simulink model "hoverSim_pid_RL"  (R2025b)
settings: Solver=ode45  StartTime=0.0  StopTime=30  RelTol=1e-3  AbsTol=1e-3  EnableMultiTasking=on
values from neighbouring files (symbols this model uses):
  A = [0 0 0 1 0 0 ... (first row only)    [setupHover.m]
  B = [0     0     0     0 ... (first row only)    [setupHover.m]
  C = [1 0 0 0 0 0 ... (first row only)    [setupHover.m]
  CMD_RATE_LIMIT = 60 * pi/180    (= 1.0471975512)    [setupHover.m]
  D = zeros(3,4)    [setupHover.m]
  K = [ 1  1  0 ... (first row only)    [setupHover.m]
  V_bias = 2.0    (= 2)    [setupHover.m]
  VMAX_AMP = 24    [setupHover.m]
  wcf = 2 * pi * 20    (= 125.663706144)    [setupHover.m]
  zetaf = 0.6    [setupHover.m]
undefined symbols (not defined in the file or in its folder): X, Y, Z
libraries: sm_lib x30, rllib x18, simulink_extras x17, slpidlib x6, nesl_utility x4, simulink x2
(part 1 of 3)
settings Model: Creator=2922887  LastModifiedBy=oleruus
settings SolverCC: AutoScaleAbsTol=off  AlgebraicLoopSolver=TrustRegion
settings DataIOCC: LimitDataPoints=on  MaxDataPoints=10000
settings OptimizationCC: LifeSpan=inf
settings DebuggingCC: UnconnectedInputMsg=warning  UnconnectedOutputMsg=warning  UnconnectedLineMsg=warning  AllowSymbolicDim=off  SFUnexpectedBacktrackingDiag=warning  SFNoUnconditionalDefaultTransitionDiag=warning  SFExecutionAtInitializationDiag=none  ArithmeticOperatorsInVariantConditions=warning
settings ModelReferenceCC: EnableRefExpFcnMdlSchedulingChecks=on
settings SFSimCC: SimUseLocalCustomCode=off  CustomCodeUndefinedFunction=UseInterfaceOnly
settings RTWCC: RTWUseLocalCustomCode=off  GPUComputeCapability=3.5  DLArmComputeVersion=19.05
settings CodeAppCC: StateflowObjectComments=on
settings GRTTargetCC: TargetLangStandard=C89/C90 (ANSI)
settings ConfigComp: CovMetricSettings=dw  CovSaveCumulativeToWorkspaceVar=on  CovSaveSingleToWorkspaceVar=on  CovExternalEMLEnable=off  CovSFcnEnable=off
settings SimscapeCC: SimscapeLogType=all  SimscapeLogSimulationStatistics=on  SimscapeLogDataHistory=10000.0
settings ExplorerConfigSet: InternalSimMechanicsExplorerSettings="<ExplorerConfiguration><canonicalview>default</canonicalview><AnimationSetting><BasePlaybackSpeed>1.0</BasePlaybackSpeed><PlaybackSpeedFactor>1.0</PlaybackSpeedFactor></AnimationSetting><TilePanel><TileInfo><Tiles Columns=\"1\" Count=\"1\" Rows=\"1\"><Column Weight=\"1\"/><Row Weight=\"1\"/><Tile Height=\"1\" Width=\"1\" X=\"0\" Y=\"0\"/></Tiles></TileInfo><SceneInfo><SceneViewer><BGColor><R>1</R><G>1</G><B>1</B></BGColor><Camera><DoPerspective>off</DoPerspective><Position><X>-0.474872206876914782</X><Y>-0.66192885214412267</Y><Z>0.674687949495536343</Z></Position><Center><X>0.0282179779907451508</X><Y>0.0797842513243843532</Y><Z>0.231109390462924141</Z></Center><Up><X>0.245225672410919443</X><Y>0.369652493337906174</Y><Z>0.896226201223598418</Z></Up><ViewLimDist>1</ViewLimDist><YLim>0.878174162375433998</YLim><XLim>0.626410921284865863</XLim></Camera></SceneViewer></SceneInfo></TilePanel><MechEditorPanel><Cameras/><GfxPanelCameraMap/><VideoCreator><PlaybackSpeedRatio>1.0</PlaybackSpeedRatio><FrameRate>30</FrameRate><VideoFormat>Motion JPEG AVI</VideoFormat><FrameSize>auto</FrameSize></VideoCreator></MechEditorPanel></ExplorerConfiguration>"

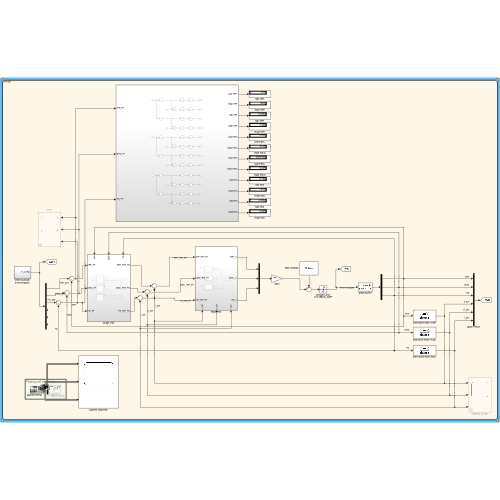
[thumbnail: Simulink's stored preview of the top-level diagram]
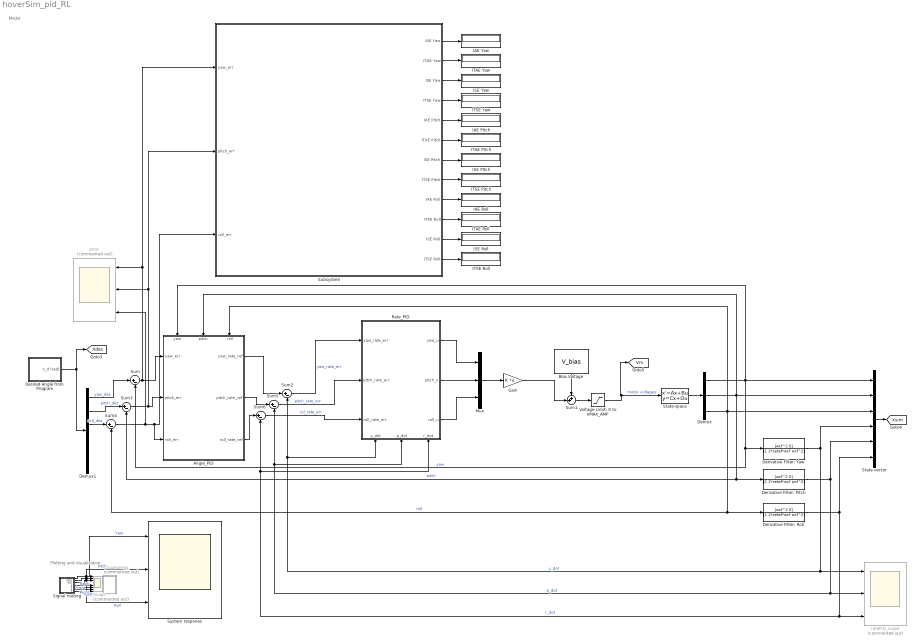
== system hoverSim_pid_RL ==
  note: Plotting and visualization
  note: Model
  Angle_PID : Subsystem
      settings: PortSchema="{\"entries\":[{\"content\":{\"sides\":[{\"content\":{\"connectorIds\":[\"In1\",\"In2\",\"In3\"]},\"type\":\"ConnectorPlacement.EquallySpacedRectSide\",\"uuid\":\"b46927c4-11e1-45df-8fc7-4aeceef11bac\"},{\"content\":{\"connectorIds\":[\"Out1\",\"Out2\",\"Out3\"],\"side\":\"RIGHT\"},\"type\":\"ConnectorPlacement.EquallySpacedRectSide\",\"uuid\":\"a6750b49-506e-4eaf-a782-8999c5d3b63d\"},{\"content\":{\"connectorIds\":[\"In4\",\"In5\",\"In6\"],\"side\":\"TOP\"},\"type\":\"ConnectorPlacement.EquallySpacedRectSide\",\"uuid\":\"43f13534-5b98-450a-b40b-fe484fdf965d\"}]},\"type\":\"ConnectorPlacement.EquallySpacedConnector\",\"uuid\":\"1f548b73-ee13-4cf6-9185-a552629201c6\"}],\"packageUris\":[\"http://schema.mathworks.com/mf0/Connector/R2020b\"],\"version\":\"1.0\"}"
  Bias Voltage : Constant  Value=V_bias
  Demux : Demux  Outputs=3
  Demux1 : Demux  Outputs=6
  Derivative Filter: Pitch : TransferFcn  Numerator=[wcf^2 0]  Denominator=[1 2*zetaf*wcf wcf^2]
  Derivative Filter: Roll : TransferFcn  Numerator=[wcf^2 0]  Denominator=[1 2*zetaf*wcf wcf^2]
  Derivative Filter: Yaw : TransferFcn  Numerator=[wcf^2 0]  Denominator=[1 2*zetaf*wcf wcf^2]
  Desired Angle from Program : Subsystem
  Gain : Gain  Gain=K  Multiplication=Matrix(K*u)
  IAE Pitch : Display
  IAE Roll : Display
  IAE Yaw : Display
  ISE Pitch : Display
  ISE Roll : Display
  ISE Yaw : Display
  ITAE Pitch : Display
  ITAE Roll : Display
  ITAE Yaw : Display
  ITSE Pitch : Display
  ITSE Roll : Display
  ITSE Yaw : Display
  Mux : Mux  Inputs=3
  Rate_PID : Subsystem
      settings: PortSchema="{\"entries\":[{\"content\":{\"sides\":[{\"content\":{\"connectorIds\":[\"In1\",\"In2\",\"In3\"]},\"type\":\"ConnectorPlacement.EquallySpacedRectSide\",\"uuid\":\"e973fd34-aa6a-4d46-8d4d-e220f6abe879\"},{\"content\":{\"connectorIds\":[\"Out1\",\"Out2\",\"Out3\"],\"side\":\"RIGHT\"},\"type\":\"ConnectorPlacement.EquallySpacedRectSide\",\"uuid\":\"8b3593b2-7102-48d7-8302-c7e837399faa\"},{\"content\":{\"side\":\"TOP\"},\"type\":\"ConnectorPlacement.EquallySpacedRectSide\",\"uuid\":\"d84d891a-66c8-41ed-b1ad-4ed19bcc84fa\"},{\"content\":{\"connectorIds\":[\"In4\",\"In5\",\"In6\"],\"side\":\"BOTTOM\"},\"type\":\"ConnectorPlacement.EquallySpacedRectSide\",\"uuid\":\"17060c95-2ed9-4508-9040-73c71d1d32f1\"}]},\"type\":\"ConnectorPlacement.EquallySpacedConnector\",\"uuid\":\"89c0bced-05a5-4749-98d6-b2176c533584\"}],\"packageUris\":[\"http://schema.mathworks.com/mf0/Connector/R2020b\"],\"version\":\"1.0\"}"
  Scope : Scope  Commented=on  NumInputPorts=8
      settings: TimeSpan=30  Title=Yaw angle  ActiveDisplayYMinimum=-0.1322186076671352  ActiveDisplayYMaximum=1.189967469004217  YLabel=deg  DataLoggingMaxPoints=10000  DataLoggingVariableName=simulationOutput
  Signal routing : Subsystem
  State vector : Mux  Inputs=6
  State-space : StateSpace  A=A  B=B  C=C  D=D  InitialCondition=0
  Subsystem : Subsystem
  Sum{,2..6} (6 alike) : Sum  Inputs=|+-
  Sum1 : Sum  Inputs=++|
  System response : Scope  NumInputPorts=3
      settings: ActiveDisplayString=3  ActiveDisplayYMinimum=-6.344757595069745  ActiveDisplayYMaximum=6.3239488034248641  YLabel=Deg  DataLoggingVariableName=ScopeData8
  Visualisering : Subsystem  Commented=on  mask{visualization=Visualization off, PacingRate=1}
      mask prompts: PacingRate "Simulation ratio (1:x) time vs real time"
      mask TypeOptions visualization: Visualization  on | Visualization off
      mask Callback visualization:
      | if get_param(append(bdroot,'/Visualisering'),'visualization') == 'Visualization  on'
      |    set_param(bdroot,'EnablePacing','on')
      | elseif get_param(append(bdroot,'/Visualisering'),'visualization') == 'Visualization off'
      |    set_param(bdroot,'EnablePacing','off')
      | end
      mask Callback PacingRate:
      | temp_param = str2num(get_param(append(bdroot,'/Visualisering'),'PacingRate'));
      | if temp_param >= 0.003 && temp_param < 0.0078
      |     set_param(bdroot,'PacingRate','0.0039')
      |     set_param(append(bdroot,'/Visualisering'),'PacingRate','0.0039')
      | elseif temp_param >= 0.0078 && temp_param < 0.0156
      |     set_param(bdroot,'PacingRate','0.0078')
      |     set_param(append(bdroot,'/Visualisering'),'PacingRate','0.0078')
      | elseif temp_param >= 0.0156 && temp_param < 0.0313
      |     set_param(bdroot,'PacingRate','0.0156')
      |     set_param(append(bdroot,'/Visualisering'),'PacingRate','0.0156')
      | elseif temp_param >= 0.0313 && temp_param < 0.0625
      |     set_param(bdroot,'PacingRate','0.0313')
      |     set_param(append(bdroot,'/Visualisering'),'PacingRate','0.0313')
      | elseif temp_param >= 0.0625 && temp_param < 0.1250
      |     set_param(bdroot,'PacingRate','0.0625')
      |     set_param(append(bdroot,'/Visualisering'),'PacingRate','0.0625')
      | elseif temp_param >= 0.1250 && temp_param < 0.2500
      |     set_param(bdroot,'PacingRate','0.1250')
      |     set_param(append(bdroot,'/Visualisering'),'PacingRate','0.1250')
      | elseif temp_param >= 0.2500 && temp_param < 0.5000
      |     set_param(bdroot, 'PacingRate','0.2500')
      |     set_param(append(bdroot,'/Visualisering'),'PacingRate','0.2500')
      | elseif temp_param >= 0.5000 && temp_param < 1
      |     set_param(bdroot, 'PacingRate','0.5000')
      |     set_param(append(bdroot,'/Visualisering'),'PacingRate','0.5000')
      | elseif temp_param >= 1 && temp_param < 2
      |     set_param(bdroot, 'PacingRate','1')
      |     set_param(append(bdroot,'/Visualisering'),'PacingRate','1')
      | elseif temp_param >= 2 && temp_param < 4
      |     set_param(bdroot, 'PacingRate','2')
      |     set_param(append(bdroot,'/Visualisering'),'PacingRate','2')
      | elseif temp_param >= 4 && temp_param < 8
      |     set_param(bdroot, 'PacingRate','4')
      |     set_param(append(bdroot,'/Visualisering'),'PacingRate','4')
      | elseif temp_param >= 8 && temp_param < 16
      |     set_param(bdroot, 'PacingRate','8')
      |     set_param(append(bdroot,'/Visualisering'),'PacingRate','8')
      | elseif temp_param >= 16 && temp_param < 32
      |     set_param(bdroot, 'PacingRate','16')
      |     set_param(append(bdroot,'/Visualisering'),'PacingRate','16')
      | elseif temp_param >= 32 && temp_param < 64
      |     set_param(bdroot, 'PacingRate','32')
      |     set_param(append(bdroot,'/Visualisering'),'PacingRate','32')
      | elseif temp_param >= 64 && temp_param < 128
      |     set_param(bdroot, 'PacingRate','64')
      |     set_param(append(bdroot,'/Visualisering'),'PacingRate','64')
      | elseif temp_param >= 128 && temp_param < 256
      |     set_param(bdroot, 'PacingRate','128')
      |     set_param(append(bdroot,'/Visualisering'),'PacingRate','128')
      | elseif temp_param >= 256
      |     set_param(bdroot, 'PacingRate','256')
      |     set_param(append(bdroot,'/Visualisering'),'PacingRate','256')
      | end
      mask DialogControl Control2 Prompt: For a 1:1 relation between the visualization model and the plotted data, the simulation ratio in this box should match the ratio in the Mechanics Explorer.
      mask DialogControl x256x Prompt: 0.0039 = 1/256x
      mask DialogControl x128x Prompt: 0.0078 = 1/128x
      mask DialogControl x64x Prompt: 0.0156 = 1/64x
      mask DialogControl x32x Prompt: 0.0313 = 1/32x
      mask DialogControl x16x Prompt: 0.0625 = 1/16x
      mask DialogControl x8x Prompt: 0.1250 = 1/8x
      mask DialogControl x4x Prompt: 0.2500 = 1/4x
      mask DialogControl x2x Prompt: 0.5000 = 1/2x
      mask Display: image('$imagefile'); % Use "Edit Image" on toolstrip to change.
  Voltage Limit: 0 to VMAX_AMP : Saturate  UpperLimit=VMAX_AMP  LowerLimit=0  LinearizeAsGain=off
  error : Scope  Commented=on  NumInputPorts=3
      settings: ActiveDisplayString=3  ActiveDisplayYMinimum=-0.22431516606316332  ActiveDisplayYMaximum=0.14053849659394291  DataLoggingVariableName=ScopeData9
  ratePID_scope : Scope  Commented=on  NumInputPorts=3
      settings: ActiveDisplayYMinimum=-0.010020272341592047  ActiveDisplayYMaximum=0.08162529177340104
  tag scope: Vm=global, Xdes=global, Xsim=global
  wires:
  Gain/1 -> Sum1/2
  Voltage Limit: 0 to VMAX_AMP/1 -> [Vm], State-space/1  "motor voltages"
  Derivative Filter: Roll/1 -> State vector/6, Sum6/2, Rate_PID/6(r_dot), ratePID_scope/3  "r_dot"
  Derivative Filter: Yaw/1 -> Sum2/2, Rate_PID/4(y_dot), ratePID_scope/1, State vector/4  "y_dot"
  State-space/1 -> Demux/1
  State vector/1 -> [Xsim]
  Demux/1 -> Angle_PID/4(yaw), State vector/1, Derivative Filter: Yaw/1, Sum/2  "yaw"
  Sum1/1 -> Voltage Limit: 0 to VMAX_AMP/1
  Bias Voltage/1 -> Sum1/1
  Demux/2 -> Angle_PID/5(pitch), State vector/2, Derivative Filter: Pitch/1, Sum3/2  "pitch"
  Derivative Filter: Pitch/1 -> State vector/5, Sum5/2, Rate_PID/5(p_dot), ratePID_scope/2  "p_dot"
  Demux/3 -> State vector/3, Angle_PID/6(roll), Derivative Filter: Roll/1, Sum4/2  "roll"
  Signal routing/1(Yaw) -> System response/1, Scope/1  "Yaw"
  Signal routing/2(Pitch) -> System response/2, Scope/2  "Pitch"
  Signal routing/3(Roll) -> System response/3, Scope/3  "Roll"
  Signal routing/4(Front motor) -> Scope/5  "Front"
  Signal routing/5(Back motor) -> Scope/6  "Back"
  Signal routing/6(Right motor) -> Scope/7  "Right"
  Signal routing/7(Left Motor) -> Scope/8  "Left"
  Desired Angle from Program/1(x_d (rad)) -> Demux1/1, [Xdes]
  Demux1/1 -> Sum/1  "yaw_des"
  Demux1/2 -> Sum3/1  "pitch_des"
  Demux1/3 -> Sum4/1  "roll_des"
  Sum2/1 -> Rate_PID/1(yaw_rate_err)  "yaw_rate_err"
  Sum5/1 -> Rate_PID/2(pitch_rate_err)  "pitch_rate_err"
  Sum6/1 -> Rate_PID/3(roll_rate_err)  "rol_rate_err"
  Rate_PID/3(roll_u) -> Mux/3
  Rate_PID/1(yaw_u) -> Mux/1
  Rate_PID/2(pitch_u) -> Mux/2
  Mux/1 -> Gain/1
  Angle_PID/1(yaw_rate_ref) -> Sum2/1
  Angle_PID/2(pitch_rate_ref) -> Sum5/1
  Angle_PID/3(roll_rate_ref) -> Sum6/1
  Sum/1 -> Subsystem/1(yaw_err), error/1, Angle_PID/1(yaw_err)
  Sum3/1 -> Subsystem/2(pitch_err), error/2, Angle_PID/2(pitch_err)
  Sum4/1 -> Angle_PID/3(roll_err), Subsystem/3(roll_err), error/3
  Subsystem/10(ITAE Roll) -> ITAE Roll/1
  Subsystem/4(ITSE Yaw) -> ITSE Yaw/1
  Subsystem/5(IAE Pitch) -> IAE Pitch/1
  Subsystem/2(ITAE Yaw) -> ITAE Yaw/1
  Subsystem/1("IAE Yaw ") -> IAE Yaw/1
  Subsystem/9(IAE Roll) -> IAE Roll/1
  Subsystem/12(ITSE Roll) -> ITSE Roll/1
  Subsystem/7(ISE Pitch) -> ISE Pitch/1
  Subsystem/8(ITSE Pitch) -> ITSE Pitch/1
  Subsystem/6(ITAE Pitch) -> ITAE Pitch/1
  Subsystem/11(ISE Roll) -> ISE Roll/1
  Subsystem/3(ISE Yaw) -> ISE Yaw/1

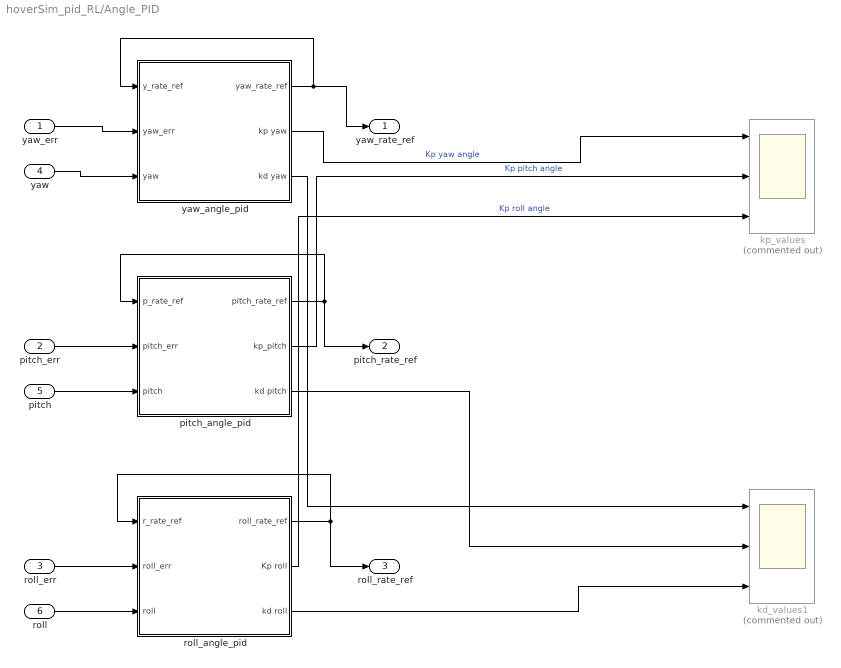
== system hoverSim_pid_RL/Angle_PID ==
  yaw_err : Inport
  pitch_err : Inport  Port=2
  roll_err : Inport  Port=3
  yaw : Inport  Port=4
  pitch : Inport  Port=5
  roll : Inport  Port=6
  kd_values1 : Scope  Commented=on  NumInputPorts=3
      settings: ActiveDisplayString=3  ActiveDisplayYMinimum=-1  ActiveDisplayYMaximum=1  YLabel=Deg  DataLoggingVariableName=ScopeData13
  kp_values : Scope  Commented=on  NumInputPorts=3
      settings: ActiveDisplayString=3  ActiveDisplayYMinimum=12.434665966429748  ActiveDisplayYMaximum=12.72289385960903  YLabel=Deg  DataLoggingVariableName=ScopeData11
  pitch_angle_pid : Subsystem
  roll_angle_pid : Subsystem
  yaw_angle_pid : Subsystem
  yaw_rate_ref : Outport
  pitch_rate_ref : Outport  Port=2
  roll_rate_ref : Outport  Port=3
  wires:
  yaw_err/1 -> yaw_angle_pid/2(yaw_err)
  pitch_err/1 -> pitch_angle_pid/2(pitch_err)
  yaw_angle_pid/1(yaw_rate_ref) -> yaw_rate_ref/1, yaw_angle_pid/1(y_rate_ref)
  pitch_angle_pid/1(pitch_rate_ref) -> pitch_rate_ref/1, pitch_angle_pid/1(p_rate_ref)
  roll_err/1 -> roll_angle_pid/2(roll_err)
  roll_angle_pid/1(roll_rate_ref) -> roll_rate_ref/1, roll_angle_pid/1(r_rate_ref)
  yaw/1 -> yaw_angle_pid/3(yaw)
  pitch/1 -> pitch_angle_pid/3(pitch)
  roll/1 -> roll_angle_pid/3(roll)
  roll_angle_pid/2(Kp roll) -> kp_values/3  "Kp roll angle"
  pitch_angle_pid/2(kp_pitch) -> kp_values/2  "Kp pitch angle"
  yaw_angle_pid/2(kp yaw) -> kp_values/1  "Kp yaw angle"
  yaw_angle_pid/3(kd yaw) -> kd_values1/1
  pitch_angle_pid/3(kd pitch) -> kd_values1/2
  roll_angle_pid/3(kd roll) -> kd_values1/3

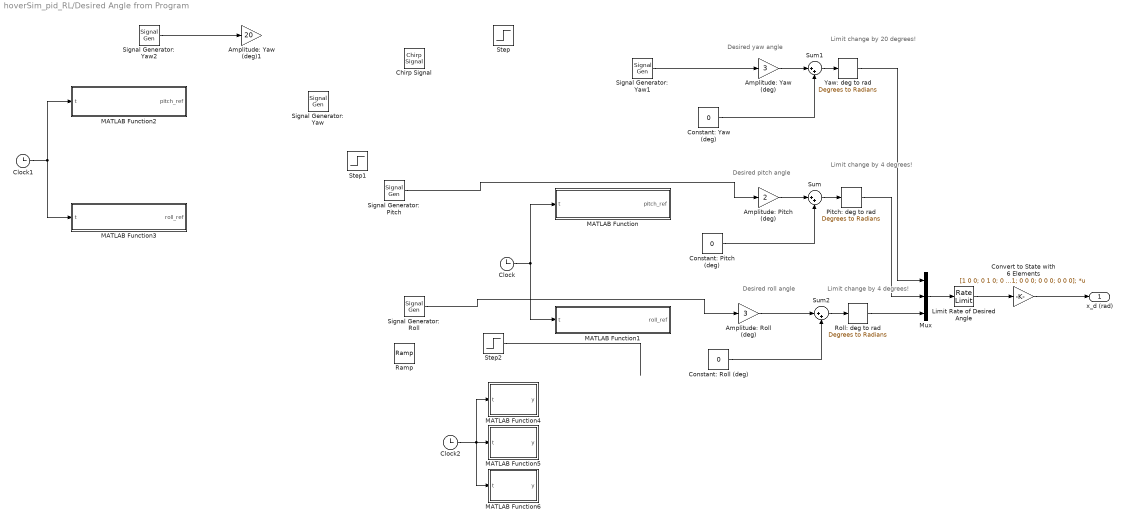
== system hoverSim_pid_RL/Desired Angle from Program ==
  note: Limit change by
      | 4 degrees!
  note: Limit change by
      | 20 degrees!
  note: Limit change by
      | 4 degrees!
  note: Desired roll angle
  note: Desired pitch angle
  note: Desired yaw angle
  Amplitude: Pitch (deg) : Gain  Gain=2
  Amplitude: Roll (deg) : Gain  Gain=3
  Amplitude: Yaw (deg) : Gain  Gain=3
  Amplitude: Yaw (deg)1 : Gain  Gain=20
  Chirp Signal : simulink/Sources/Chirp Signal  f1=0.1  T=30  f2=0.7
  Clock : Clock
  Clock1 : Clock
  Clock2 : Clock
  Constant: Pitch (deg) : Constant  Value=0
  Constant: Roll (deg) : Constant  Value=0
  Constant: Yaw (deg) : Constant  Value=0
  Convert to State with 6 Elements : Gain  Gain=[1 0 0; 0 1 0; 0 0 1; 0 0 0; 0 0 0; 0 0 0];  Multiplication=Matrix(K*u)
  Limit Rate of Desired Angle : RateLimiter  RisingSlewLimit=CMD_RATE_LIMIT  FallingSlewLimit=-CMD_RATE_LIMIT
  MATLAB Function : MATLAB Function  TreatAsAtomicUnit=on
  MATLAB Function1 : MATLAB Function  TreatAsAtomicUnit=on
  MATLAB Function2 : MATLAB Function  TreatAsAtomicUnit=on
  MATLAB Function3 : MATLAB Function  TreatAsAtomicUnit=on
  MATLAB Function4 : MATLAB Function  TreatAsAtomicUnit=on
  MATLAB Function5 : MATLAB Function  TreatAsAtomicUnit=on
  MATLAB Function6 : MATLAB Function  TreatAsAtomicUnit=on
  Mux : Mux  Inputs=3
  Pitch: deg to rad : simulink_extras/Transformations/Degrees to Radians
  Ramp : simulink/Sources/Ramp  slope=3  start=3  InitialOutput=0
  Roll: deg to rad : simulink_extras/Transformations/Degrees to Radians
  Signal Generator: Pitch : SignalGenerator  Amplitude=6  Frequency=0.06
  Signal Generator: Roll : SignalGenerator  WaveForm=square  Frequency=0.08
  Signal Generator: Yaw : SignalGenerator  Amplitude=5  Frequency=0.1
  Signal Generator: Yaw1 : SignalGenerator  WaveForm=square  Frequency=0.06
  Signal Generator: Yaw2 : SignalGenerator  WaveForm=square  Frequency=0.06
  Step : Step  Time=2  SampleTime=0
  Step1 : Step  Time=5  SampleTime=0
  Step2 : Step  Time=8  SampleTime=0
  Sum : Sum  Inputs=|++
  Sum1 : Sum  Inputs=|++
  Sum2 : Sum  Inputs=|++
  Yaw: deg to rad : simulink_extras/Transformations/Degrees to Radians
  x_d (rad) : Outport
  wires:
  Convert to State with 6 Elements/1 -> x_d (rad)/1
  Limit Rate of Desired Angle/1 -> Convert to State with 6 Elements/1
  Roll: deg to rad/1 -> Mux/3
  Pitch: deg to rad/1 -> Mux/2
  Yaw: deg to rad/1 -> Mux/1
  Sum2/1 -> Roll: deg to rad/1
  Constant: Roll (deg)/1 -> Sum2/2
  Sum/1 -> Pitch: deg to rad/1
  Constant: Pitch (deg)/1 -> Sum/2
  Sum1/1 -> Yaw: deg to rad/1
  Amplitude: Yaw (deg)/1 -> Sum1/1
  Constant: Yaw (deg)/1 -> Sum1/2
  Mux/1 -> Limit Rate of Desired Angle/1
  Clock/1 -> MATLAB Function/1(t), MATLAB Function1/1(t)
  Clock1/1 -> MATLAB Function2/1(t), MATLAB Function3/1(t)
  Signal Generator: Yaw2/1 -> Amplitude: Yaw (deg)1/1
  Clock2/1 -> MATLAB Function6/1(t), MATLAB Function4/1(t), MATLAB Function5/1(t)
  Amplitude: Pitch (deg)/1 -> Sum/1
  Amplitude: Roll (deg)/1 -> Sum2/1
  Signal Generator: Pitch/1 -> Amplitude: Pitch (deg)/1
  Signal Generator: Yaw1/1 -> Amplitude: Yaw (deg)/1
  Step2/1 -> ?
  Signal Generator: Roll/1 -> Amplitude: Roll (deg)/1

== system hoverSim_pid_RL/Rate_PID ==
  yaw_rate_err : Inport
  pitch_rate_err : Inport  Port=2
  roll_rate_err : Inport  Port=3
  y_dot : Inport  Port=4
  p_dot : Inport  Port=5
  r_dot : Inport  Port=6
  ki_values1 : Scope  Commented=on  NumInputPorts=3
      settings: ActiveDisplayString=3  ActiveDisplayYMinimum=-1  ActiveDisplayYMaximum=1  YLabel=Deg  DataLoggingVariableName=ScopeData12
  pitch_rate_pid : Subsystem
  roll_rate_pid : Subsystem
  yaw_rate_pid : Subsystem
  yaw_u : Outport
  pitch_u : Outport  Port=2
  roll_u : Outport  Port=3
  wires:
  pitch_rate_err/1 -> pitch_rate_pid/1(pitch_rate_err)
  pitch_rate_pid/1(pitch_rate_ref) -> pitch_rate_pid/3(u_p), pitch_u/1
  yaw_rate_err/1 -> yaw_rate_pid/1(yaw_rate_err)
  yaw_rate_pid/1(yaw_rate_ref) -> yaw_rate_pid/3(u_y), yaw_u/1
  roll_rate_pid/1(roll_rate_ref) -> roll_rate_pid/3(u_r), roll_u/1
  roll_rate_err/1 -> roll_rate_pid/1(roll_rate_err)
  y_dot/1 -> yaw_rate_pid/2(y_dot)
  p_dot/1 -> pitch_rate_pid/2(p_dot)
  r_dot/1 -> roll_rate_pid/2(r_dot)
  yaw_rate_pid/2(ki_rate) -> ki_values1/1  "ki yaw"
  pitch_rate_pid/2(ki_rate) -> ki_values1/2  "ki pitch"
  roll_rate_pid/2(ki_rate) -> ki_values1/3  "ki roll"

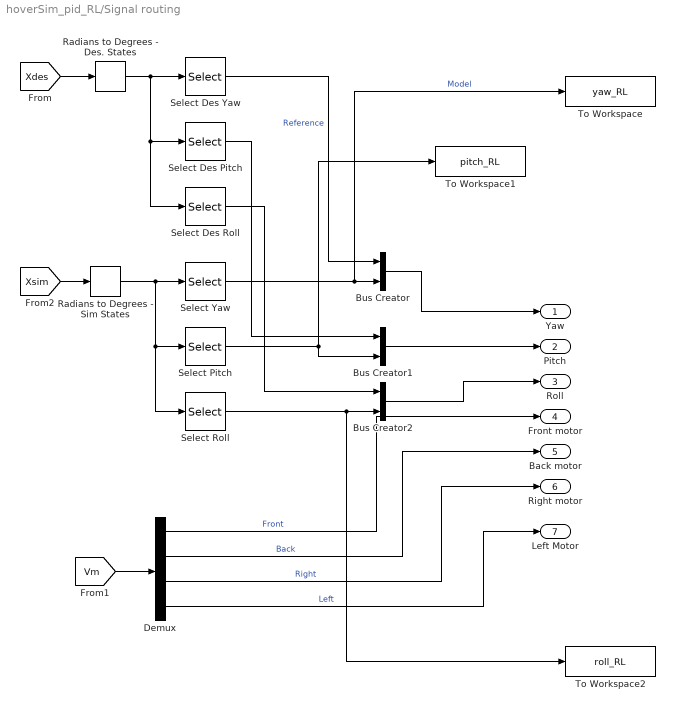
== system hoverSim_pid_RL/Signal routing ==
  Bus Creator : BusCreator  Inputs=2
  Bus Creator1 : BusCreator  Inputs=2
  Bus Creator2 : BusCreator  Inputs=2
  Demux : Demux
  Radians to Degrees - Des. States : simulink_extras/Transformations/Radians to Degrees
  Radians to Degrees - Sim States : simulink_extras/Transformations/Radians to Degrees
  Select Des Pitch : Selector  InputPortWidth=6  IndexOptions=Index vector (dialog)  Indices=2  OutputSizes=1
  Select Des Roll : Selector  InputPortWidth=6  IndexOptions=Index vector (dialog)  Indices=3  OutputSizes=1
  Select Des Yaw : Selector  InputPortWidth=6  IndexOptions=Index vector (dialog)  Indices=1  OutputSizes=1
  Select Pitch : Selector  InputPortWidth=6  IndexOptions=Index vector (dialog)  Indices=2  OutputSizes=1
  Select Roll : Selector  InputPortWidth=6  IndexOptions=Index vector (dialog)  Indices=3  OutputSizes=1
  Select Yaw : Selector  InputPortWidth=6  IndexOptions=Index vector (dialog)  Indices=1  OutputSizes=1
  To Workspace : ToWorkspace  VariableName=yaw_RL  SaveFormat=Timeseries  SampleTime=-1
  To Workspace1 : ToWorkspace  VariableName=pitch_RL  SaveFormat=Timeseries  SampleTime=-1
  To Workspace2 : ToWorkspace  VariableName=roll_RL  SaveFormat=Timeseries  SampleTime=-1
  Yaw : Outport
  Pitch : Outport  Port=2
  Roll : Outport  Port=3
  Front motor : Outport  Port=4
  Back motor : Outport  Port=5
  Right motor : Outport  Port=6
  Left Motor : Outport  Port=7
  wires:
  Select Des Roll/1 -> Bus Creator2/1
  Select Des Yaw/1 -> Bus Creator/1  "Reference"
  Radians to Degrees - Des. States/1 -> Select Des Roll/1, Select Des Pitch/1, Select Des Yaw/1
  Select Roll/1 -> To Workspace2/1, Bus Creator2/2
  Select Pitch/1 -> To Workspace1/1, Bus Creator1/2
  Select Yaw/1 -> To Workspace/1, Bus Creator/2  "Model"
  Bus Creator2/1 -> Roll/1
  Radians to Degrees - Sim States/1 -> Select Roll/1, Select Pitch/1, Select Yaw/1
  Bus Creator1/1 -> Pitch/1
  Bus Creator/1 -> Yaw/1
  [Xsim] -> Radians to Degrees - Sim States/1
  [Xdes] -> Radians to Degrees - Des. States/1
  [Vm] -> Demux/1
  Demux/1 -> Front motor/1  "Front"
  Demux/2 -> Back motor/1  "Back"
  Demux/3 -> Right motor/1  "Right"
  Demux/4 -> Left Motor/1  "Left"
  Select Des Pitch/1 -> Bus Creator1/1

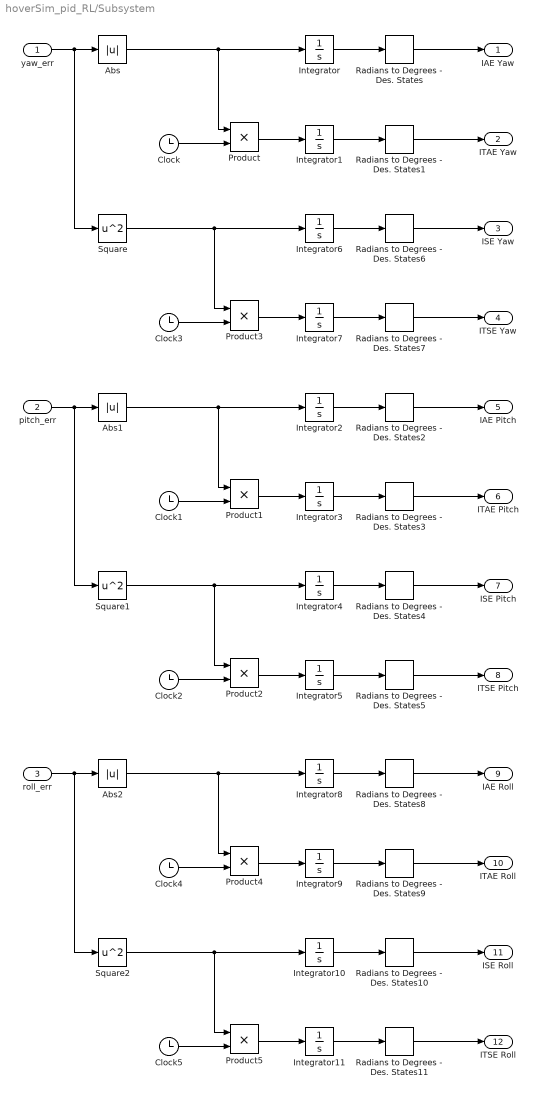
== system hoverSim_pid_RL/Subsystem ==
  yaw_err : Inport
  pitch_err : Inport  Port=2
  roll_err : Inport  Port=3
  Abs : Abs  SaturateOnIntegerOverflow=off
  Abs1 : Abs  SaturateOnIntegerOverflow=off
  Abs2 : Abs  SaturateOnIntegerOverflow=off
  Clock{,1..5} (6 alike) : Clock
  Integrator{,1..11} (12 alike) : Integrator
  Product{,1..5} (6 alike) : Product
  Radians to Degrees - Des. States{,1..11} (12 alike) : simulink_extras/Transformations/Radians to Degrees
  Square : Math  Operator=square
  Square1 : Math  Operator=square
  Square2 : Math  Operator=square
  "IAE Yaw " : Outport
  ITAE Yaw : Outport  Port=2
  ISE Yaw : Outport  Port=3
  ITSE Yaw : Outport  Port=4
  IAE Pitch : Outport  Port=5
  ITAE Pitch : Outport  Port=6
  ISE Pitch : Outport  Port=7
  ITSE Pitch : Outport  Port=8
  IAE Roll : Outport  Port=9
  ITAE Roll : Outport  Port=10
  ISE Roll : Outport  Port=11
  ITSE Roll : Outport  Port=12
  wires:
  yaw_err/1 -> Abs/1, Square/1
  Clock/1 -> Product/2
  Abs/1 -> Integrator/1, Product/1
  Product/1 -> Integrator1/1
  Integrator/1 -> Radians to Degrees - Des. States/1
  Integrator1/1 -> Radians to Degrees - Des. States1/1
  Square/1 -> Product3/1, Integrator6/1
  Clock3/1 -> Product3/2
  Product3/1 -> Integrator7/1
  Integrator7/1 -> Radians to Degrees - Des. States7/1
  Integrator6/1 -> Radians to Degrees - Des. States6/1
  Radians to Degrees - Des. States/1 -> "IAE Yaw "/1
  Radians to Degrees - Des. States1/1 -> ITAE Yaw/1
  Radians to Degrees - Des. States6/1 -> ISE Yaw/1
  Radians to Degrees - Des. States7/1 -> ITSE Yaw/1
  Clock1/1 -> Product1/2
  Radians to Degrees - Des. States5/1 -> ITSE Pitch/1
  Clock2/1 -> Product2/2
  Product1/1 -> Integrator3/1
  Integrator3/1 -> Radians to Degrees - Des. States3/1
  Abs1/1 -> Integrator2/1, Product1/1
  Integrator2/1 -> Radians to Degrees - Des. States2/1
  pitch_err/1 -> Abs1/1, Square1/1
  Integrator5/1 -> Radians to Degrees - Des. States5/1
  Integrator4/1 -> Radians to Degrees - Des. States4/1
  Radians to Degrees - Des. States4/1 -> ISE Pitch/1
  Product2/1 -> Integrator5/1
  Square1/1 -> Product2/1, Integrator4/1
  Radians to Degrees - Des. States3/1 -> ITAE Pitch/1
  Radians to Degrees - Des. States2/1 -> IAE Pitch/1
  Clock4/1 -> Product4/2
  Radians to Degrees - Des. States11/1 -> ITSE Roll/1
  Clock5/1 -> Product5/2
  Product4/1 -> Integrator9/1
  Integrator9/1 -> Radians to Degrees - Des. States9/1
  Abs2/1 -> Integrator8/1, Product4/1
  Integrator8/1 -> Radians to Degrees - Des. States8/1
  roll_err/1 -> Abs2/1, Square2/1
  Integrator11/1 -> Radians to Degrees - Des. States11/1
  Integrator10/1 -> Radians to Degrees - Des. States10/1
  Radians to Degrees - Des. States10/1 -> ISE Roll/1
  Product5/1 -> Integrator11/1
  Square2/1 -> Product5/1, Integrator10/1
  Radians to Degrees - Des. States9/1 -> ITAE Roll/1
  Radians to Degrees - Des. States8/1 -> IAE Roll/1

== system hoverSim_pid_RL/Visualisering ==
  Constant : Constant  Value=visualization
  Constant1 : Constant
  Constant2 : Constant  Value=-1
  Demux : Demux  Outputs=3
  Display : Display
  Enabled Subsystem : Subsystem  TreatAsAtomicUnit=on
  Selector : Selector  InputPortWidth=6  IndexOptions=Index vector (dialog)  Indices=[1 2 3]  OutputSizes=1
  Switch : Switch  Criteria=u2 > Threshold  Threshold=1  SaturateOnIntegerOverflow=off  InputSameDT=off
  wires:
  Constant1/1 -> Switch/3
  Constant2/1 -> Switch/1
  Switch/1 -> Enabled Subsystem/Enable
  Constant/1 -> Display/1, Switch/2
  [Xsim] -> Selector/1
  Selector/1 -> Demux/1
  Demux/1 -> Enabled Subsystem/1(yaw)
  Demux/2 -> Enabled Subsystem/2(pitch)
  Demux/3 -> Enabled Subsystem/3(roll)

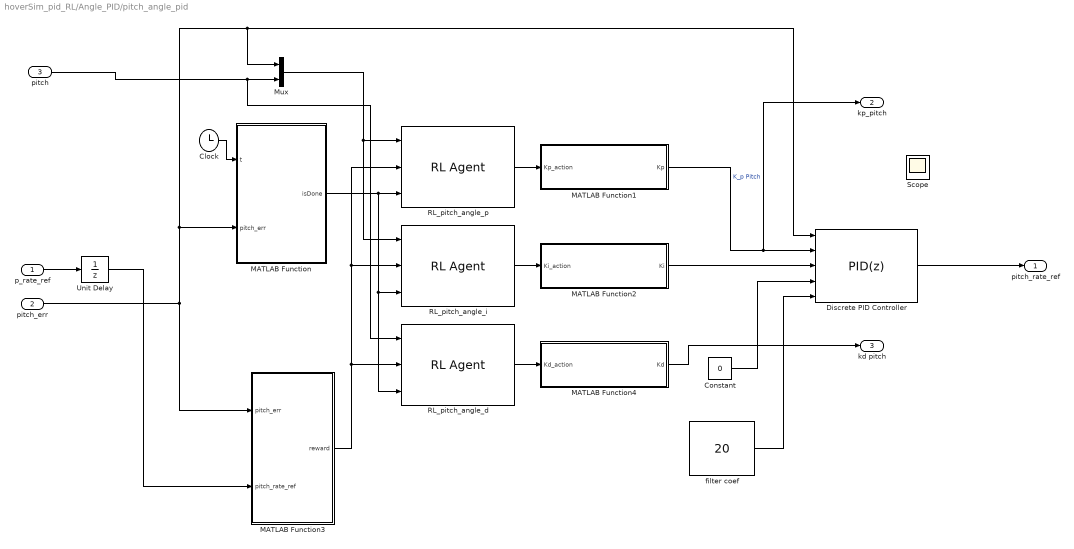
== system hoverSim_pid_RL/Angle_PID/pitch_angle_pid ==
  p_rate_ref : Inport
  pitch_err : Inport  Port=2
  pitch : Inport  Port=3
  Clock : Clock
  Constant : Constant  Value=0
  Discrete PID Controller : slpidlib/PID Controller  Controller=PID  Form=Parallel  TimeDomain=Discrete-time  UseExternalTs=off  SampleTime=-1  IntegratorMethod=Forward Euler  FilterMethod=Forward Euler  ControllerParametersSource=external  P=1  I=1  UseKiTs=off  D=0  UseExternalDerivativeSource=off  N=100  UseFilter=on  TunerSelectOption=Transfer Function Based (PID Tuner App)  InitialConditionSource=internal  InitialConditionForIntegrator=0  InitialConditionForFilter=0  DifferentiatorICPrevScaledInput=0  ExternalReset=none  TrackingMode=off  Kt=1  LimitOutput=off  SatLimitsSource=internal  UpperSaturationLimit=inf  LowerSaturationLimit=-inf  LinearizeAsGain=off  AntiWindupMode=none  Kb=1  LimitIntegrator=off  UpperIntegratorSaturationLimit=inf  LowerIntegratorSaturationLimit=-inf  POutMin=[]  POutMax=[]  IOutMin=[]  IOutMax=[]  DOutMin=[]  DOutMax=[]  NOutMin=[]  NOutMax=[]  SumOutMin=[]  SumOutMax=[]  SaturationOutMin=[]  SaturationOutMax=[]  PParamMin=[]  PParamMax=[]  IParamMin=[]  IParamMax=[]  DParamMin=[]  DParamMax=[]  NParamMin=[]  NParamMax=[]  KbParamMin=[]  KbParamMax=[]  KtParamMin=[]  KtParamMax=[]  KbOutMin=[]  KbOutMax=[]  KtOutMin=[]  KtOutMax=[]  IntegratorOutMin=[]  IntegratorOutMax=[]  FilterOutMin=[]  FilterOutMax=[]  SumI1OutMin=[]  SumI1OutMax=[]  SumI2OutMin=[]  SumI2OutMax=[]  SumI3OutMin=[]  SumI3OutMax=[]  SumI4OutMin=[]  SumI4OutMax=[]  SumDOutMin=[]  SumDOutMax=[]  DifferentiatorOutMin=[]  DifferentiatorOutMax=[]  FilterDiffOutCoefMin=[]  FilterDiffOutCoefMax=[]  ReciprocalOutMin=[]  ReciprocalOutMax=[]  SumDenOutMin=[]  SumDenOutMax=[]  SumNumOutMin=[]  SumNumOutMax=[]  DivideOutMin=[]  DivideOutMax=[]  UdiffTsProdOutMin=[]  UdiffTsProdOutMax=[]  NTsProdOutMin=[]  NTsProdOutMax=[]  UintegralTsProdOutMin=[]  UintegralTsProdOutMax=[]  UngainTsProdOutMin=[]  UngainTsProdOutMax=[]  ClampingZeroOutDataTypeStr=Inherit: Inherit via back propagation  ClampingZeroOutMin=[]  ClampingZeroOutMax=[]  FilterDenConstantOutDataTypeStr=Inherit: Inherit via back propagation  FilterDenConstantOutMin=[]  FilterDenConstantOutMax=[]  PCopyOutDataTypeStr=Inherit: Inherit via back propagation  PCopyOutMin=[]  PCopyOutMax=[]  NCopyOutDataTypeStr=Inherit: Inherit via back propagation  NCopyOutMin=[]  NCopyOutMax=[]  IntegratorContinuousStateAttributes=''  IntegratorStateMustResolveToSignalObject=off  IntegratorRTWStateStorageClass=Auto  FilterContinuousStateAttributes=''  FilterStateMustResolveToSignalObject=off  FilterRTWStateStorageClass=Auto  ParallelPVariant=ExternalParameters  IdealPVariant=Disabled  IVariant=ExternalParameters  DVariant=ExternalParameters  IntegratorVariant=Discrete  SatVariant=Disabled  AWVariant=Passthrough  PCopyVariant=Disabled  TRVariant=Disabled  FdbkBlocksVariant=Forward  IdealPFdbkVariant=Disabled  SatFdbkVariant=Disabled  DerivativeFilterVariant=ForwardEulerFilter  NVariant=ExternalParameters  NCopyVariant=Disabled  FilterICVariant=InternalICsFilter  IntegratorICVariant=InternalICs  ExternalResetVariant=Disabled  TRSumVariant=Passthrough  SumFdbkVariant=Disabled  SumVariant=Sum_PID  TsampFilterVariant=InternalTs  TsampNgainVariant=Passthrough  TsampIntegralVariant=Disabled_SignalSpec  ExternalSaturationOutDataTypeStr=Inherit: Same as second input  DerivativeSourceVariant=ErrorSignal  PreIntVariant=InternalPreInt
      settings: LibrarySourceBlock=simulink/Discrete/Discrete PID Controller
  MATLAB Function : MATLAB Function  TreatAsAtomicUnit=on
  MATLAB Function1 : MATLAB Function  TreatAsAtomicUnit=on
  MATLAB Function2 : MATLAB Function  TreatAsAtomicUnit=on
  MATLAB Function3 : MATLAB Function  TreatAsAtomicUnit=on
  MATLAB Function4 : MATLAB Function  TreatAsAtomicUnit=on
  Mux : Mux  Inputs=2
  RL_pitch_angle_d : rllib/RL Agent  Agent=pitch_angle_d  ExternalActionAsInput=off  ProvideLastAction=off  ProvideCumRwd=off  TreatAsDirectFeedthrough=on  UseStrictObservationDataTypes=off
  RL_pitch_angle_i : rllib/RL Agent  Agent=pitch_angle_i  ExternalActionAsInput=off  ProvideLastAction=off  ProvideCumRwd=off  TreatAsDirectFeedthrough=on  UseStrictObservationDataTypes=off
  RL_pitch_angle_p : rllib/RL Agent  Agent=pitch_angle_p  ExternalActionAsInput=off  ProvideLastAction=off  ProvideCumRwd=off  TreatAsDirectFeedthrough=on  UseStrictObservationDataTypes=off
  Scope : Scope
      settings: DataLoggingVariableName=ScopeData10
  Unit Delay : UnitDelay  SampleTime=-1  HasFrameUpgradeWarning=on
  filter coef : Constant  Value=20
  pitch_rate_ref : Outport
  kp_pitch : Outport  Port=2
  kd pitch : Outport  Port=3
  wires:
  filter coef/1 -> Discrete PID Controller/5
  RL_pitch_angle_p/1 -> MATLAB Function1/1(Kp_action)
  RL_pitch_angle_i/1 -> MATLAB Function2/1(Ki_action)
  RL_pitch_angle_d/1 -> MATLAB Function4/1(Kd_action)
  pitch_err/1 -> MATLAB Function3/1(pitch_err), Mux/1, Discrete PID Controller/1, MATLAB Function/2(pitch_err)
  Clock/1 -> MATLAB Function/1(t)
  MATLAB Function3/1(reward) -> RL_pitch_angle_d/2, RL_pitch_angle_i/2, RL_pitch_angle_p/2
  MATLAB Function/1(isDone) -> RL_pitch_angle_p/3, RL_pitch_angle_i/3, RL_pitch_angle_d/3
  p_rate_ref/1 -> Unit Delay/1
  Constant/1 -> Discrete PID Controller/4
  Discrete PID Controller/1 -> pitch_rate_ref/1
  pitch/1 -> RL_pitch_angle_d/1, Mux/2
  Mux/1 -> RL_pitch_angle_i/1, RL_pitch_angle_p/1
  MATLAB Function1/1(Kp) -> kp_pitch/1, Discrete PID Controller/2  "K_p Pitch"
  Unit Delay/1 -> MATLAB Function3/2(pitch_rate_ref)
  MATLAB Function4/1(Kd) -> kd pitch/1
  MATLAB Function2/1(Ki) -> Discrete PID Controller/3

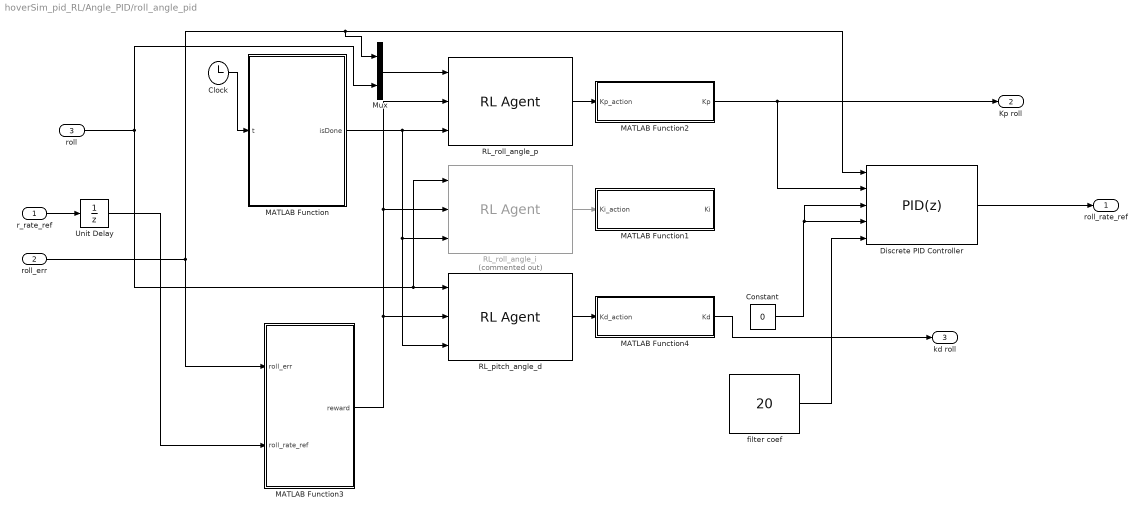
== system hoverSim_pid_RL/Angle_PID/roll_angle_pid ==
  r_rate_ref : Inport
  roll_err : Inport  Port=2
  roll : Inport  Port=3
  Clock : Clock
  Constant : Constant  Value=0
  Discrete PID Controller : slpidlib/PID Controller  Controller=PID  Form=Parallel  TimeDomain=Discrete-time  UseExternalTs=off  SampleTime=-1  IntegratorMethod=Forward Euler  FilterMethod=Forward Euler  ControllerParametersSource=external  P=1  I=1  UseKiTs=off  D=0  UseExternalDerivativeSource=off  N=100  UseFilter=on  TunerSelectOption=Transfer Function Based (PID Tuner App)  InitialConditionSource=internal  InitialConditionForIntegrator=0  InitialConditionForFilter=0  DifferentiatorICPrevScaledInput=0  ExternalReset=none  TrackingMode=off  Kt=1  LimitOutput=off  SatLimitsSource=internal  UpperSaturationLimit=inf  LowerSaturationLimit=-inf  LinearizeAsGain=off  AntiWindupMode=none  Kb=1  LimitIntegrator=off  UpperIntegratorSaturationLimit=inf  LowerIntegratorSaturationLimit=-inf  POutMin=[]  POutMax=[]  IOutMin=[]  IOutMax=[]  DOutMin=[]  DOutMax=[]  NOutMin=[]  NOutMax=[]  SumOutMin=[]  SumOutMax=[]  SaturationOutMin=[]  SaturationOutMax=[]  PParamMin=[]  PParamMax=[]  IParamMin=[]  IParamMax=[]  DParamMin=[]  DParamMax=[]  NParamMin=[]  NParamMax=[]  KbParamMin=[]  KbParamMax=[]  KtParamMin=[]  KtParamMax=[]  KbOutMin=[]  KbOutMax=[]  KtOutMin=[]  KtOutMax=[]  IntegratorOutMin=[]  IntegratorOutMax=[]  FilterOutMin=[]  FilterOutMax=[]  SumI1OutMin=[]  SumI1OutMax=[]  SumI2OutMin=[]  SumI2OutMax=[]  SumI3OutMin=[]  SumI3OutMax=[]  SumI4OutMin=[]  SumI4OutMax=[]  SumDOutMin=[]  SumDOutMax=[]  DifferentiatorOutMin=[]  DifferentiatorOutMax=[]  FilterDiffOutCoefMin=[]  FilterDiffOutCoefMax=[]  ReciprocalOutMin=[]  ReciprocalOutMax=[]  SumDenOutMin=[]  SumDenOutMax=[]  SumNumOutMin=[]  SumNumOutMax=[]  DivideOutMin=[]  DivideOutMax=[]  UdiffTsProdOutMin=[]  UdiffTsProdOutMax=[]  NTsProdOutMin=[]  NTsProdOutMax=[]  UintegralTsProdOutMin=[]  UintegralTsProdOutMax=[]  UngainTsProdOutMin=[]  UngainTsProdOutMax=[]  ClampingZeroOutDataTypeStr=Inherit: Inherit via back propagation  ClampingZeroOutMin=[]  ClampingZeroOutMax=[]  FilterDenConstantOutDataTypeStr=Inherit: Inherit via back propagation  FilterDenConstantOutMin=[]  FilterDenConstantOutMax=[]  PCopyOutDataTypeStr=Inherit: Inherit via back propagation  PCopyOutMin=[]  PCopyOutMax=[]  NCopyOutDataTypeStr=Inherit: Inherit via back propagation  NCopyOutMin=[]  NCopyOutMax=[]  IntegratorContinuousStateAttributes=''  IntegratorStateMustResolveToSignalObject=off  IntegratorRTWStateStorageClass=Auto  FilterContinuousStateAttributes=''  FilterStateMustResolveToSignalObject=off  FilterRTWStateStorageClass=Auto  ParallelPVariant=ExternalParameters  IdealPVariant=Disabled  IVariant=ExternalParameters  DVariant=ExternalParameters  IntegratorVariant=Discrete  SatVariant=Disabled  AWVariant=Passthrough  PCopyVariant=Disabled  TRVariant=Disabled  FdbkBlocksVariant=Forward  IdealPFdbkVariant=Disabled  SatFdbkVariant=Disabled  DerivativeFilterVariant=ForwardEulerFilter  NVariant=ExternalParameters  NCopyVariant=Disabled  FilterICVariant=InternalICsFilter  IntegratorICVariant=InternalICs  ExternalResetVariant=Disabled  TRSumVariant=Passthrough  SumFdbkVariant=Disabled  SumVariant=Sum_PID  TsampFilterVariant=InternalTs  TsampNgainVariant=Passthrough  TsampIntegralVariant=Disabled_SignalSpec  ExternalSaturationOutDataTypeStr=Inherit: Same as second input  DerivativeSourceVariant=ErrorSignal  PreIntVariant=InternalPreInt
      settings: LibrarySourceBlock=simulink/Discrete/Discrete PID Controller
  MATLAB Function : MATLAB Function  TreatAsAtomicUnit=on
  MATLAB Function1 : MATLAB Function  TreatAsAtomicUnit=on
  MATLAB Function2 : MATLAB Function  TreatAsAtomicUnit=on
  MATLAB Function3 : MATLAB Function  TreatAsAtomicUnit=on
  MATLAB Function4 : MATLAB Function  TreatAsAtomicUnit=on
  Mux : Mux  Inputs=2
  RL_pitch_angle_d : rllib/RL Agent  Agent=pitch_angle_d  ExternalActionAsInput=off  ProvideLastAction=off  ProvideCumRwd=off  TreatAsDirectFeedthrough=on  UseStrictObservationDataTypes=off
  RL_roll_angle_i : rllib/RL Agent  Commented=on  Agent=roll_angle_i  ExternalActionAsInput=off  ProvideLastAction=off  ProvideCumRwd=off  TreatAsDirectFeedthrough=on  UseStrictObservationDataTypes=off
  RL_roll_angle_p : rllib/RL Agent  Agent=roll_angle_p  ExternalActionAsInput=off  ProvideLastAction=off  ProvideCumRwd=off  TreatAsDirectFeedthrough=on  UseStrictObservationDataTypes=off
  Unit Delay : UnitDelay  SampleTime=-1  HasFrameUpgradeWarning=on
  filter coef : Constant  Value=20
  roll_rate_ref : Outport
  Kp roll : Outport  Port=2
  kd roll : Outport  Port=3
  wires:
  filter coef/1 -> Discrete PID Controller/5
  Constant/1 -> Discrete PID Controller/3, Discrete PID Controller/4
  RL_roll_angle_p/1 -> MATLAB Function2/1(Kp_action)
  RL_roll_angle_i/1 -> MATLAB Function1/1(Ki_action)
  RL_pitch_angle_d/1 -> MATLAB Function4/1(Kd_action)
  Unit Delay/1 -> MATLAB Function3/2(roll_rate_ref)
  roll_err/1 -> Mux/1, Discrete PID Controller/1, MATLAB Function3/1(roll_err)
  Clock/1 -> MATLAB Function/1(t)
  MATLAB Function3/1(reward) -> RL_pitch_angle_d/2, RL_roll_angle_i/2, RL_roll_angle_p/2
  MATLAB Function/1(isDone) -> RL_roll_angle_p/3, RL_pitch_angle_d/3, RL_roll_angle_i/3
  r_rate_ref/1 -> Unit Delay/1
  Discrete PID Controller/1 -> roll_rate_ref/1
  MATLAB Function2/1(Kp) -> Kp roll/1, Discrete PID Controller/2
  Mux/1 -> RL_roll_angle_p/1
  roll/1 -> Mux/2, RL_roll_angle_i/1, RL_pitch_angle_d/1
  MATLAB Function4/1(Kd) -> kd roll/1

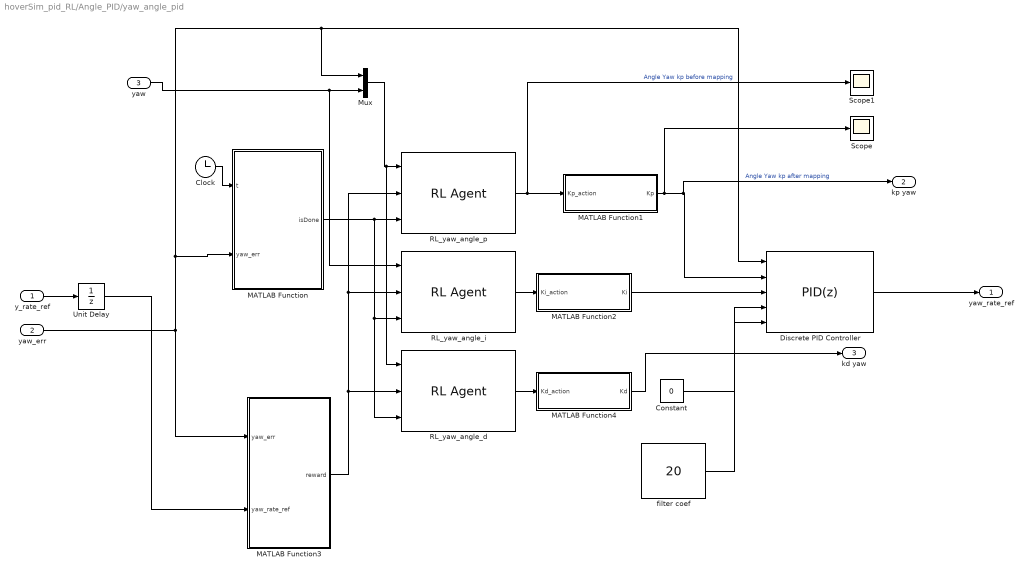
== system hoverSim_pid_RL/Angle_PID/yaw_angle_pid ==
  y_rate_ref : Inport
  yaw_err : Inport  Port=2
  yaw : Inport  Port=3
  Clock : Clock
  Constant : Constant  Value=0
  Discrete PID Controller : slpidlib/PID Controller  Controller=PID  Form=Parallel  TimeDomain=Discrete-time  UseExternalTs=off  SampleTime=-1  IntegratorMethod=Forward Euler  FilterMethod=Forward Euler  ControllerParametersSource=external  P=1  I=1  UseKiTs=off  D=0  UseExternalDerivativeSource=off  N=100  UseFilter=on  TunerSelectOption=Transfer Function Based (PID Tuner App)  InitialConditionSource=internal  InitialConditionForIntegrator=0  InitialConditionForFilter=0  DifferentiatorICPrevScaledInput=0  ExternalReset=none  TrackingMode=off  Kt=1  LimitOutput=off  SatLimitsSource=internal  UpperSaturationLimit=inf  LowerSaturationLimit=-inf  LinearizeAsGain=off  AntiWindupMode=none  Kb=1  LimitIntegrator=off  UpperIntegratorSaturationLimit=inf  LowerIntegratorSaturationLimit=-inf  POutMin=[]  POutMax=[]  IOutMin=[]  IOutMax=[]  DOutMin=[]  DOutMax=[]  NOutMin=[]  NOutMax=[]  SumOutMin=[]  SumOutMax=[]  SaturationOutMin=[]  SaturationOutMax=[]  PParamMin=[]  PParamMax=[]  IParamMin=[]  IParamMax=[]  DParamMin=[]  DParamMax=[]  NParamMin=[]  NParamMax=[]  KbParamMin=[]  KbParamMax=[]  KtParamMin=[]  KtParamMax=[]  KbOutMin=[]  KbOutMax=[]  KtOutMin=[]  KtOutMax=[]  IntegratorOutMin=[]  IntegratorOutMax=[]  FilterOutMin=[]  FilterOutMax=[]  SumI1OutMin=[]  SumI1OutMax=[]  SumI2OutMin=[]  SumI2OutMax=[]  SumI3OutMin=[]  SumI3OutMax=[]  SumI4OutMin=[]  SumI4OutMax=[]  SumDOutMin=[]  SumDOutMax=[]  DifferentiatorOutMin=[]  DifferentiatorOutMax=[]  FilterDiffOutCoefMin=[]  FilterDiffOutCoefMax=[]  ReciprocalOutMin=[]  ReciprocalOutMax=[]  SumDenOutMin=[]  SumDenOutMax=[]  SumNumOutMin=[]  SumNumOutMax=[]  DivideOutMin=[]  DivideOutMax=[]  UdiffTsProdOutMin=[]  UdiffTsProdOutMax=[]  NTsProdOutMin=[]  NTsProdOutMax=[]  UintegralTsProdOutMin=[]  UintegralTsProdOutMax=[]  UngainTsProdOutMin=[]  UngainTsProdOutMax=[]  ClampingZeroOutDataTypeStr=Inherit: Inherit via back propagation  ClampingZeroOutMin=[]  ClampingZeroOutMax=[]  FilterDenConstantOutDataTypeStr=Inherit: Inherit via back propagation  FilterDenConstantOutMin=[]  FilterDenConstantOutMax=[]  PCopyOutDataTypeStr=Inherit: Inherit via back propagation  PCopyOutMin=[]  PCopyOutMax=[]  NCopyOutDataTypeStr=Inherit: Inherit via back propagation  NCopyOutMin=[]  NCopyOutMax=[]  IntegratorContinuousStateAttributes=''  IntegratorStateMustResolveToSignalObject=off  IntegratorRTWStateStorageClass=Auto  FilterContinuousStateAttributes=''  FilterStateMustResolveToSignalObject=off  FilterRTWStateStorageClass=Auto  ParallelPVariant=ExternalParameters  IdealPVariant=Disabled  IVariant=ExternalParameters  DVariant=ExternalParameters  IntegratorVariant=Discrete  SatVariant=Disabled  AWVariant=Passthrough  PCopyVariant=Disabled  TRVariant=Disabled  FdbkBlocksVariant=Forward  IdealPFdbkVariant=Disabled  SatFdbkVariant=Disabled  DerivativeFilterVariant=ForwardEulerFilter  NVariant=ExternalParameters  NCopyVariant=Disabled  FilterICVariant=InternalICsFilter  IntegratorICVariant=InternalICs  ExternalResetVariant=Disabled  TRSumVariant=Passthrough  SumFdbkVariant=Disabled  SumVariant=Sum_PID  TsampFilterVariant=InternalTs  TsampNgainVariant=Passthrough  TsampIntegralVariant=Disabled_SignalSpec  ExternalSaturationOutDataTypeStr=Inherit: Same as second input  DerivativeSourceVariant=ErrorSignal  PreIntVariant=InternalPreInt
      settings: LibrarySourceBlock=simulink/Discrete/Discrete PID Controller
  MATLAB Function : MATLAB Function  TreatAsAtomicUnit=on
  MATLAB Function1 : MATLAB Function  TreatAsAtomicUnit=on
  MATLAB Function2 : MATLAB Function  TreatAsAtomicUnit=on
  MATLAB Function3 : MATLAB Function  TreatAsAtomicUnit=on
  MATLAB Function4 : MATLAB Function  TreatAsAtomicUnit=on
  Mux : Mux  Inputs=2
  RL_yaw_angle_d : rllib/RL Agent  Agent=yaw_angle_d  ExternalActionAsInput=off  ProvideLastAction=off  ProvideCumRwd=off  TreatAsDirectFeedthrough=on  UseStrictObservationDataTypes=off
  RL_yaw_angle_i : rllib/RL Agent  Agent=yaw_angle_i  ExternalActionAsInput=off  ProvideLastAction=off  ProvideCumRwd=off  TreatAsDirectFeedthrough=on  UseStrictObservationDataTypes=off
  RL_yaw_angle_p : rllib/RL Agent  Agent=yaw_angle_p  ExternalActionAsInput=off  ProvideLastAction=off  ProvideCumRwd=off  TreatAsDirectFeedthrough=on  UseStrictObservationDataTypes=off
  Scope : Scope
      settings: ActiveDisplayYMinimum=-1  ActiveDisplayYMaximum=1  YLabel=K_p Yaw angle  DataLoggingVariableName=ScopeData6
  Scope1 : Scope
      settings: ActiveDisplayYMinimum=-0.31677602827548978  ActiveDisplayYMaximum=-0.1167760282754898  YLabel=RL agent action  DataLoggingVariableName=ScopeData7
  Unit Delay : UnitDelay  SampleTime=-1  HasFrameUpgradeWarning=on
  filter coef : Constant  Value=20
  yaw_rate_ref : Outport
  kp yaw : Outport  Port=2
  kd yaw : Outport  Port=3
  wires:
  filter coef/1 -> Discrete PID Controller/5
  yaw_err/1 -> MATLAB Function3/1(yaw_err), MATLAB Function/2(yaw_err), Mux/1, Discrete PID Controller/1
  RL_yaw_angle_p/1 -> Scope1/1, MATLAB Function1/1(Kp_action)  "Angle Yaw kp before mapping"
  RL_yaw_angle_i/1 -> MATLAB Function2/1(Ki_action)
  RL_yaw_angle_d/1 -> MATLAB Function4/1(Kd_action)
  MATLAB Function/1(isDone) -> RL_yaw_angle_p/3, RL_yaw_angle_d/3, RL_yaw_angle_i/3
  y_rate_ref/1 -> Unit Delay/1
  MATLAB Function3/1(reward) -> RL_yaw_angle_p/2, RL_yaw_angle_i/2, RL_yaw_angle_d/2
  Clock/1 -> MATLAB Function/1(t)
  Unit Delay/1 -> MATLAB Function3/2(yaw_rate_ref)
  Discrete PID Controller/1 -> yaw_rate_ref/1
  MATLAB Function1/1(Kp) -> Scope/1, kp yaw/1, Discrete PID Controller/2  "Angle Yaw kp after mapping"
  yaw/1 -> RL_yaw_angle_i/1, Mux/2
  Mux/1 -> RL_yaw_angle_p/1, RL_yaw_angle_d/1
  MATLAB Function4/1(Kd) -> kd yaw/1
  MATLAB Function2/1(Ki) -> Discrete PID Controller/3
  Constant/1 -> Discrete PID Controller/4

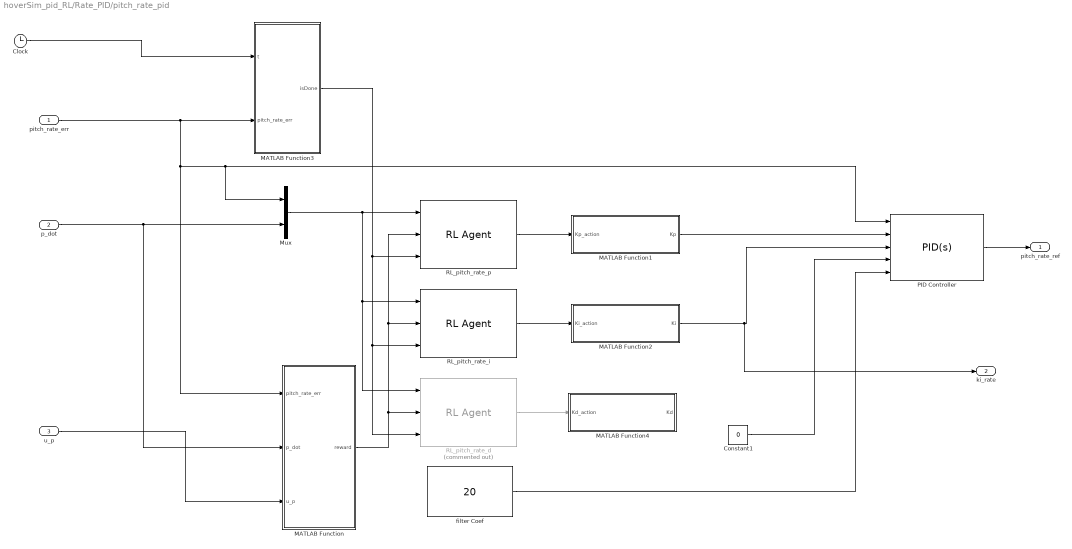
== system hoverSim_pid_RL/Rate_PID/pitch_rate_pid ==
  pitch_rate_err : Inport
  p_dot : Inport  Port=2
  u_p : Inport  Port=3
  Clock : Clock
  Constant1 : Constant  Value=0
  MATLAB Function : MATLAB Function  TreatAsAtomicUnit=on
  MATLAB Function1 : MATLAB Function  TreatAsAtomicUnit=on
  MATLAB Function2 : MATLAB Function  TreatAsAtomicUnit=on
  MATLAB Function3 : MATLAB Function  TreatAsAtomicUnit=on
  MATLAB Function4 : MATLAB Function  TreatAsAtomicUnit=on
  Mux : Mux  Inputs=2
  PID Controller : slpidlib/PID Controller  Controller=PID  Form=Parallel  TimeDomain=Continuous-time  UseExternalTs=off  SampleTime=-1  IntegratorMethod=Forward Euler  FilterMethod=Forward Euler  ControllerParametersSource=external  P=1  I=1  UseKiTs=off  D=0  UseExternalDerivativeSource=off  N=100  UseFilter=on  TunerSelectOption=Transfer Function Based (PID Tuner App)  InitialConditionSource=internal  InitialConditionForIntegrator=0  InitialConditionForFilter=0  DifferentiatorICPrevScaledInput=0  ExternalReset=none  TrackingMode=off  Kt=1  LimitOutput=off  SatLimitsSource=internal  UpperSaturationLimit=inf  LowerSaturationLimit=-inf  LinearizeAsGain=on  AntiWindupMode=none  Kb=1  LimitIntegrator=off  UpperIntegratorSaturationLimit=inf  LowerIntegratorSaturationLimit=-inf  POutMin=[]  POutMax=[]  IOutMin=[]  IOutMax=[]  DOutMin=[]  DOutMax=[]  NOutMin=[]  NOutMax=[]  SumOutMin=[]  SumOutMax=[]  SaturationOutMin=[]  SaturationOutMax=[]  PParamMin=[]  PParamMax=[]  IParamMin=[]  IParamMax=[]  DParamMin=[]  DParamMax=[]  NParamMin=[]  NParamMax=[]  KbParamMin=[]  KbParamMax=[]  KtParamMin=[]  KtParamMax=[]  KbOutMin=[]  KbOutMax=[]  KtOutMin=[]  KtOutMax=[]  IntegratorOutMin=[]  IntegratorOutMax=[]  FilterOutMin=[]  FilterOutMax=[]  SumI1OutMin=[]  SumI1OutMax=[]  SumI2OutMin=[]  SumI2OutMax=[]  SumI3OutMin=[]  SumI3OutMax=[]  SumI4OutMin=[]  SumI4OutMax=[]  SumDOutMin=[]  SumDOutMax=[]  DifferentiatorOutMin=[]  DifferentiatorOutMax=[]  FilterDiffOutCoefMin=[]  FilterDiffOutCoefMax=[]  ReciprocalOutMin=[]  ReciprocalOutMax=[]  SumDenOutMin=[]  SumDenOutMax=[]  SumNumOutMin=[]  SumNumOutMax=[]  DivideOutMin=[]  DivideOutMax=[]  UdiffTsProdOutMin=[]  UdiffTsProdOutMax=[]  NTsProdOutMin=[]  NTsProdOutMax=[]  UintegralTsProdOutMin=[]  UintegralTsProdOutMax=[]  UngainTsProdOutMin=[]  UngainTsProdOutMax=[]  ClampingZeroOutDataTypeStr=Inherit: Inherit via back propagation  ClampingZeroOutMin=[]  ClampingZeroOutMax=[]  FilterDenConstantOutDataTypeStr=Inherit: Inherit via back propagation  FilterDenConstantOutMin=[]  FilterDenConstantOutMax=[]  PCopyOutDataTypeStr=Inherit: Inherit via back propagation  PCopyOutMin=[]  PCopyOutMax=[]  NCopyOutDataTypeStr=Inherit: Inherit via back propagation  NCopyOutMin=[]  NCopyOutMax=[]  IntegratorContinuousStateAttributes=''  IntegratorStateMustResolveToSignalObject=off  IntegratorRTWStateStorageClass=Auto  FilterContinuousStateAttributes=''  FilterStateMustResolveToSignalObject=off  FilterRTWStateStorageClass=Auto  ParallelPVariant=ExternalParameters  IdealPVariant=Disabled  IVariant=ExternalParameters  DVariant=ExternalParameters  IntegratorVariant=Continuous  SatVariant=Disabled  AWVariant=Passthrough  PCopyVariant=Disabled  TRVariant=Disabled  FdbkBlocksVariant=Forward  IdealPFdbkVariant=Disabled  SatFdbkVariant=Disabled  DerivativeFilterVariant=ContFilter  NVariant=ExternalParameters  NCopyVariant=Disabled  FilterICVariant=InternalICsFilter  IntegratorICVariant=InternalICs  ExternalResetVariant=Disabled  TRSumVariant=Passthrough  SumFdbkVariant=Disabled  SumVariant=Sum_PID  TsampFilterVariant=InternalTs  TsampNgainVariant=Passthrough  TsampIntegralVariant=Disabled_SignalSpec  ExternalSaturationOutDataTypeStr=Inherit: Same as second input  DerivativeSourceVariant=ErrorSignal  PreIntVariant=InternalPreInt
  RL_pitch_rate_d : rllib/RL Agent  Commented=on  Agent=pitch_rate_d  ExternalActionAsInput=off  ProvideLastAction=off  ProvideCumRwd=off  TreatAsDirectFeedthrough=on  UseStrictObservationDataTypes=off
  RL_pitch_rate_i : rllib/RL Agent  Agent=pitch_rate_i  ExternalActionAsInput=off  ProvideLastAction=off  ProvideCumRwd=off  TreatAsDirectFeedthrough=on  UseStrictObservationDataTypes=off
  RL_pitch_rate_p : rllib/RL Agent  Agent=pitch_rate_p  ExternalActionAsInput=off  ProvideLastAction=off  ProvideCumRwd=off  TreatAsDirectFeedthrough=on  UseStrictObservationDataTypes=off
  filter Coef : Constant  Value=20
  pitch_rate_ref : Outport
  ki_rate : Outport  Port=2
  wires:
  PID Controller/1 -> pitch_rate_ref/1
  filter Coef/1 -> PID Controller/5
  MATLAB Function/1(reward) -> RL_pitch_rate_d/2, RL_pitch_rate_i/2, RL_pitch_rate_p/2
  p_dot/1 -> MATLAB Function/2(p_dot), Mux/2
  u_p/1 -> MATLAB Function/3(u_p)
  Clock/1 -> MATLAB Function3/1(t)
  MATLAB Function3/1(isDone) -> RL_pitch_rate_p/3, RL_pitch_rate_d/3, RL_pitch_rate_i/3
  pitch_rate_err/1 -> MATLAB Function/1(pitch_rate_err), Mux/1, PID Controller/1, MATLAB Function3/2(pitch_rate_err)
  RL_pitch_rate_p/1 -> MATLAB Function1/1(Kp_action)
  RL_pitch_rate_d/1 -> MATLAB Function4/1(Kd_action)
  RL_pitch_rate_i/1 -> MATLAB Function2/1(Ki_action)
  Constant1/1 -> PID Controller/4
  MATLAB Function1/1(Kp) -> PID Controller/2
  Mux/1 -> RL_pitch_rate_d/1, RL_pitch_rate_i/1, RL_pitch_rate_p/1
  MATLAB Function2/1(Ki) -> ki_rate/1, PID Controller/3
